simulink model "subsysChanged"  (R2024b)
settings: Solver=VariableStepAuto  StartTime=0.0  StopTime=10.0  RelTol=1e-3
settings Model: Creator=neham
settings RTWCC: GPUComputeCapability=3.5

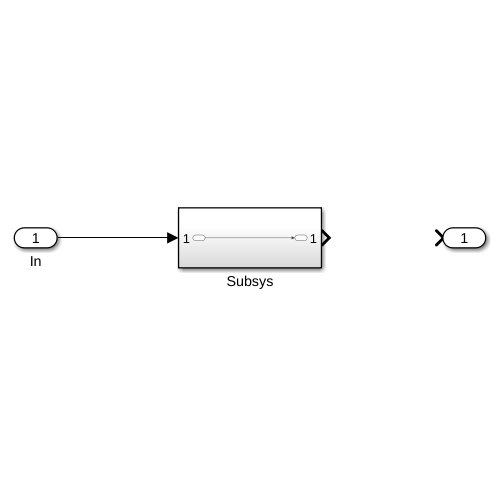
[thumbnail: Simulink's stored preview of the top-level diagram]
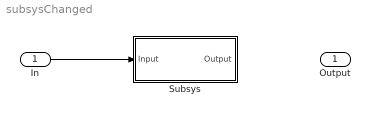
== system subsysChanged ==
  In : Inport
  Subsys : Subsystem
  Output : Outport
  wires:
  In/1 -> Subsys/1(Input)

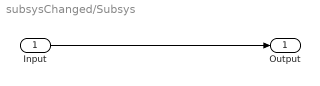
== system subsysChanged/Subsys ==
  Input : Inport
  Output : Outport
  wires:
  Input/1 -> Output/1
